simulink model "Timestamp"  (R2020a)
settings: Solver=FixedStepAuto  StartTime=0.0  StopTime=10.0  FixedStep=1e-3  RelTol=1e-3  EnableMultiTasking=on
libraries: frdmk64flib x1
settings Model: ExtModeTrigDuration=5  Creator=WinnieTrandinh  LastModifiedBy=WinnieTrandinh
settings OptimizationCC: EnhancedBackFolding=on  PassReuseOutputArgsAs=Individual arguments  ZeroExternalMemoryAtStartup=off  ZeroInternalMemoryAtStartup=off  MaxStackSize=64  OptimizeBlockOrder=speed  DifferentSizesBufferReuse=on  OptimizationCustomize=off  EfficientTunableParamExpr=on
settings DebuggingCC: ParameterTunabilityLossMsg=error
settings HardwareCC: ProdBitPerPointer=32  ProdBitPerSizeT=32  ProdBitPerPtrDiffT=32  ProdLargestAtomicInteger=Long  ProdLargestAtomicFloat=Double  ProdWordSize=32  ProdHWDeviceType=ARM Compatible->ARM Cortex
settings SFSimCC: MATLABDynamicMemAlloc=off
settings RTWCC: SystemTargetFile=ert.tlc  HardwareBoard=NXP FRDM-K64F  TemplateMakefile=ert_default_tmf  Toolchain=GNU Tools for ARM Embedded Processors
settings CodeAppCC: ForceParamTrailComments=on  IgnoreCustomStorageClasses=off  OperatorAnnotations=on  SimulinkDataObjDesc=on  SFDataObjDesc=on  InsertBlockDesc=on

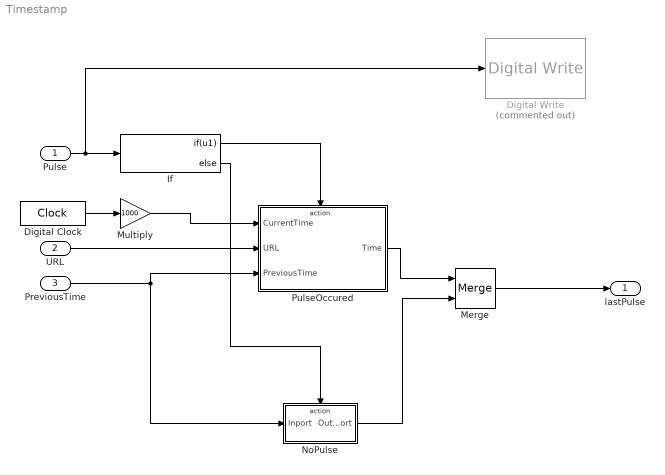
== system Timestamp ==
  Pulse : Inport  OutDataTypeStr=boolean
  URL : Inport  Port=2  Unit=ms
  PreviousTime : Inport  Port=3
  Digital Clock : DigitalClock  SampleTime=0.001
  Digital Write : frdmk64flib/Digital Write  Commented=on  Whichpin=GREEN_LED
  If : If  IfExpression=u1
  Merge : Merge
  Multiply : Gain  Gain=1000
  NoPulse : Subsystem  TreatAsAtomicUnit=on
  PulseOccured : Subsystem  TreatAsAtomicUnit=on
  lastPulse : Outport
  wires:
  If/2 -> NoPulse/Action
  NoPulse/1(Outport) -> Merge/2
  Digital Clock/1 -> Multiply/1
  PulseOccured/1(Time) -> Merge/1
  If/1 -> PulseOccured/Action
  Merge/1 -> lastPulse/1
  Multiply/1 -> PulseOccured/1(CurrentTime)
  URL/1 -> PulseOccured/2(URL)
  PreviousTime/1 -> NoPulse/1(Inport), PulseOccured/3(PreviousTime)
  Pulse/1 -> Digital Write/1, If/1

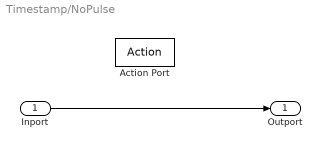
== system Timestamp/NoPulse ==
  Inport : Inport
  Action Port : ActionPort  ActionPortLabel=else
  Outport : Outport
  wires:
  Inport/1 -> Outport/1

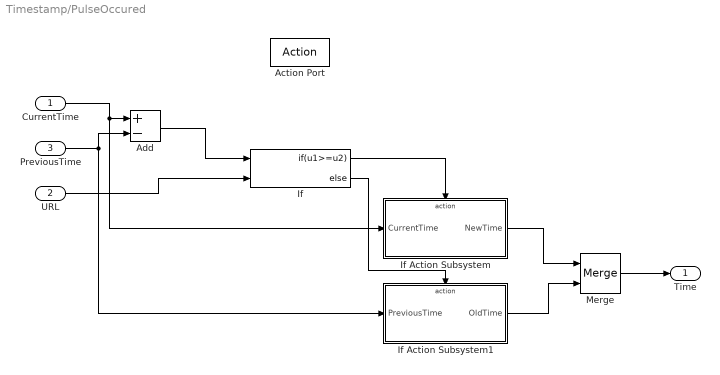
== system Timestamp/PulseOccured ==
  CurrentTime : Inport
  URL : Inport  Port=2
  PreviousTime : Inport  Port=3
  Action Port : ActionPort  ActionPortLabel=if(u1)
  Add : Sum  Inputs=+-
  If : If  NumInputs=2  IfExpression=u1>=u2
  If Action Subsystem : Subsystem  TreatAsAtomicUnit=on
  If Action Subsystem1 : Subsystem  TreatAsAtomicUnit=on
  Merge : Merge
  Time : Outport
  wires:
  CurrentTime/1 -> Add/1, If Action Subsystem/1(CurrentTime)
  PreviousTime/1 -> If Action Subsystem1/1(PreviousTime), Add/2
  Add/1 -> If/1
  URL/1 -> If/2
  If/1 -> If Action Subsystem/Action
  Merge/1 -> Time/1
  If Action Subsystem/1(NewTime) -> Merge/1
  If Action Subsystem1/1(OldTime) -> Merge/2
  If/2 -> If Action Subsystem1/Action

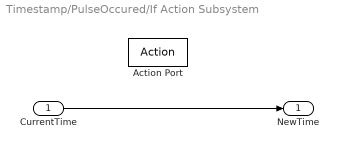
== system Timestamp/PulseOccured/If Action Subsystem ==
  CurrentTime : Inport
  Action Port : ActionPort  ActionPortLabel=if(u1>=u2)
  NewTime : Outport
  wires:
  CurrentTime/1 -> NewTime/1

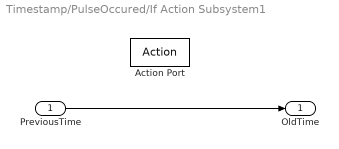
== system Timestamp/PulseOccured/If Action Subsystem1 ==
  PreviousTime : Inport
  Action Port : ActionPort  ActionPortLabel=else
  OldTime : Outport
  wires:
  PreviousTime/1 -> OldTime/1
